simulink model "mldemo_suspn"  (Simulink 6.6)
settings: Solver=ode45  SolverMode=SingleTasking  StartTime=0.0  StopTime=10  MaxStep=0.01  RelTol=1e-3  AbsTol=1e-6
StopFcn:
  | pause(0.1)
  | mldemo_suspgraph
model workspace: external: M-Code (data not in the file)
values from neighbouring files (symbols this model uses):
  cf = cf0    (= 2200)    [configParams.m]    (also in myCostFcn.m = x(2); myCostFcnRR.m = x(2); mynonlcon.m = x(2); mynonlconRR.m = x(2))
  cr = cr0    (= 2000)    [configParams.m]    (also in myCostFcn.m = x(4); myCostFcnRR.m = x(4); mynonlcon.m = x(4); mynonlconRR.m = x(4))
  Iyy = Iyyempty    (= 2100)    [configParams.m]    (also in tweakmymass.m = Iyy1 - Mb*cm^2)
  kf = kf0    (= 19600)    [configParams.m]    (also in myCostFcn.m = x(1); myCostFcnRR.m = x(1); mynonlcon.m = x(1); mynonlconRR.m = x(1))
  kr = kr0    (= 14700)    [configParams.m]    (also in myCostFcn.m = x(3); myCostFcnRR.m = x(3); mynonlcon.m = x(3); mynonlconRR.m = x(3))
  Lf = Lf0    (= 0.9)    [configParams.m]    (also in tweakmymass.m = Lf0 - cm)
  Lr = Lr0    (= 1.2)    [configParams.m]    (also in tweakmymass.m = Lr0 + cm)
  Mb = Mempty    (= 1200)    [configParams.m]    (also in tweakmymass.m = Mempty + front + back + trunk)
  theta0 = 0    [configParams.m]
  thetadot0 = 0    [configParams.m]
  Z0 = -0.5*Mb*g/(kf+kr)    (= -0.171603498542)    [configParams.m]
  Zdot0 = 0    [configParams.m]
Description:
  | Automotive Suspension
  | 
  | This demo describes a simplified half-car model that includes an independent
  | front and rear vertical suspension. The model also includes body pitch and
  | bounce degrees of freedom. The demo provides a description of the model to
  | show how simulation can be used for investigating ride characteristics.
  | In conjunction with a powertrain simulation, the model could
  | investigate longitudinal shuffle resulting from changes in throttle setting.
settings Model: Creator=The MathWorks Inc.  LastModifiedBy=tschultz  ExtModeTrigMode=oneshot  ExtModeArmWhenConnect=off  ExtModeAutoUpdateStatusClock=off
settings DataIOCC: InitialState=x0  LimitDataPoints=off  SaveFormat=StructureWithTime  SaveOutput=off  StateSaveName=x  TimeSaveName=t  SignalLoggingName=sldemo_suspn_output
settings OptimizationCC: BooleanDataType=off  InlineInvariantSignals=on  BufferReusableBoundary=off
settings DebuggingCC: SignalResolutionControl=TryResolveAllWithWarning  SolverPrmCheckMsg=none  MultiTaskDSMMsg=warning  SigSpecEnsureSampleTimeMsg=none  IntegerOverflowMsg=none  BusObjectLabelMismatch=none  StrictBusMsg=ErrorLevel1
settings HardwareCC: TargetUnknown=on
settings RTWCC: IncludeERTFirstTime=on

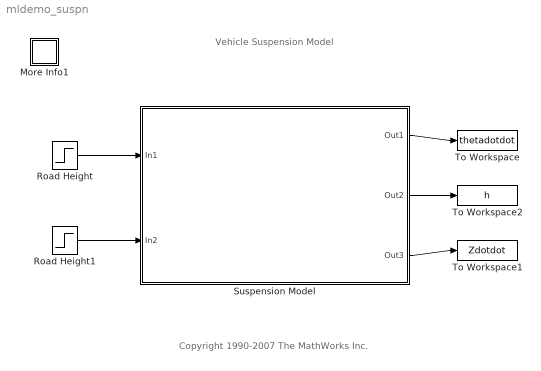
== system mldemo_suspn ==
  note: Vehicle Suspension Model
  note: Copyright 1990-2007 The MathWorks Inc.
  More Info1 : Subsystem
      settings: OpenFcn=showdemo(bdroot(gcb))
      mask Display: disp('?')
  Road Height : Step  After=0.01  SampleTime=0
  Road Height1 : Step  Time=2  After=-0.01  SampleTime=0
  Suspension Model : Subsystem
      mask Display: plot(-1, 0, 13, 12, [1 12], [11 11], [1 5], [2 2], [1 2], [4.5 5], [2 0], [5 6], [0 2], [6 7], [2 0], [7 8], [0 1], [8 8.5], [1 1], [8.5 11], [1 1], [2 4.5], [5 5], [2 5], [4 6], [5 5], [4 4], [5 8], [6 6], [5 8], [4 6], [6.5 6.5], [5 5], [6.5 11], [0 1], [1 2], [2 3], [1 2], [4 5], [1 2])
  To Workspace : ToWorkspace  VariableName=thetadotdot  SampleTime=-1  SaveFormat=Array
  To Workspace1 : ToWorkspace  VariableName=Zdotdot  SampleTime=-1  SaveFormat=Array
  To Workspace2 : ToWorkspace  VariableName=h  SampleTime=-1  SaveFormat=Array
  wires:
  Road Height/1 -> Suspension Model/1(In1)
  Road Height1/1 -> Suspension Model/2(In2)
  Suspension Model/1(Out1) -> To Workspace/1
  Suspension Model/2(Out2) -> To Workspace2/1
  Suspension Model/3(Out3) -> To Workspace1/1

== system mldemo_suspn/More Info1 ==

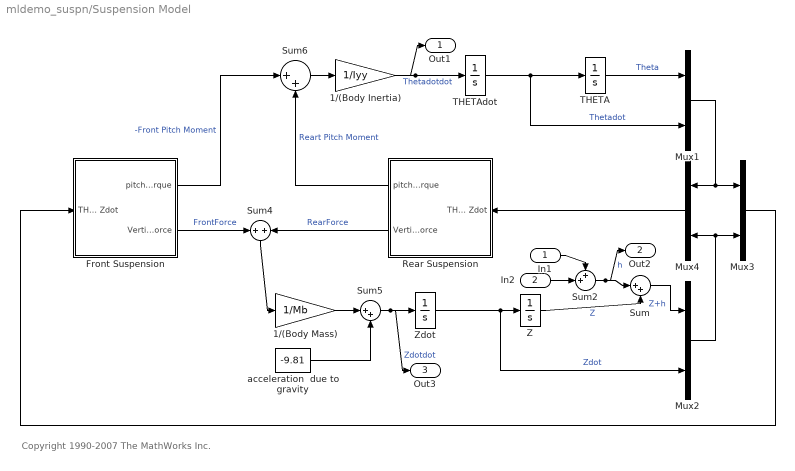
== system mldemo_suspn/Suspension Model ==
  note: Copyright 1990-2007 The MathWorks Inc.
  In1 : Inport
  In2 : Inport  Port=2
  1/(Body Inertia) : Gain  Gain=1/Iyy  SaturateOnIntegerOverflow=on
  1/(Body Mass) : Gain  Gain=1/Mb  SaturateOnIntegerOverflow=on
  Front Suspension : Subsystem  mask(half-car suspension){K=kf, C=cf, L=-Lf}
      mask prompts: K "Stiffness = spring rate:"; C "Damping rate:"; L "Moment arm:"
      mask help:
      | Half-Car Suspension
      | The spring and damping rates for an individual wheel are entered below.  Their combined effect as applied to two wheels at the specified distance from the center of mass is computed.  The distance should be specified as positive if the subsystem is oriented such that increasing z corresponds to increasing theta, negative otherwise.
      mask Help: See "Using Simulink and Stateflow in Automotive Applications" for a mathematical derivation of the subsystem operation.  Contact your MathWorks distributor to obtain a copy.
      mask Display: plot(-1, 0, 13, 12, [1 12], [11 11], [1 5], [2 2], [1 2], [4.5 5], [2 0], [5 6], [0 2], [6 7], [2 0], [7 8], [0 1], [8 8.5], [1 1], [8.5 11], [1 1], [2 4.5], [5 5], [2 5], [4 6], [5 5], [4 4], [5 8], [6 6], [5 8], [4 6], [6.5 6.5], [5 5], [6.5 11], [0 1], [1 2], [2 3], [1 2], [4 5], [1 2])
  Mux1 : Mux  Inputs=2
      settings: DisplayOption=signals
  Mux2 : Mux  Inputs=2
      settings: DisplayOption=signals
  Mux3 : Mux  Inputs=2
      settings: DisplayOption=signals
  Mux4 : Mux  Orientation=left  Inputs=2
      settings: DisplayOption=signals
  Rear Suspension : Subsystem  Orientation=left  mask(half-car suspension){K=kr, C=cr, L=Lr}
      mask prompts: K "Stiffness = spring rate:"; C "Damping rate:"; L "Moment arm:"
      mask help:
      | Half-Car Suspension
      | The spring and damping rates for an individual wheel are entered below.  Their combined effect as applied to two wheels at the specified distance from the center of mass is computed.  The distance should be specified as positive if the subsystem is oriented such that increasing z corresponds to increasing theta, negative otherwise.
      mask Help: See "Using Simulink and Stateflow in Automotive Applications" for a mathematical derivation of the subsystem operation.  Contact your MathWorks distributor to obtain a copy.
      mask Display: plot(-1, 0, 13, 12, [1 12], [11 11], [1 5], [2 2], [1 2], [4.5 5], [2 0], [5 6], [0 2], [6 7], [2 0], [7 8], [0 1], [8 8.5], [1 1], [8.5 11], [1 1], [2 4.5], [5 5], [2 5], [4 6], [5 5], [4 4], [5 8], [6 6], [5 8], [4 6], [6.5 6.5], [5 5], [6.5 11], [0 1], [1 2], [2 3], [1 2], [4 5], [1 2])
  Sum : Sum  Inputs=|++
  Sum2 : Sum  Inputs=++|
  Sum4 : Sum  Orientation=down  SaturateOnIntegerOverflow=on  InputSameDT=on
  Sum5 : Sum  Inputs=|++  SaturateOnIntegerOverflow=on  InputSameDT=on
  Sum6 : Sum  Inputs=|++  SaturateOnIntegerOverflow=on  InputSameDT=on
  THETA : Integrator  InitialCondition=theta0  ContinuousStateAttributes='theta'
  THETAdot : Integrator  InitialCondition=thetadot0  ContinuousStateAttributes='thetadot'
  Z : Integrator  InitialCondition=Z0  ContinuousStateAttributes='Z'
  Zdot : Integrator  InitialCondition=Zdot0  ContinuousStateAttributes='Zdot'
  acceleration  due to gravity : Constant  Value=-9.81
  Out1 : Outport
  Out2 : Outport  Port=2
  Out3 : Outport  Port=3
  wires:
  Front Suspension/2(Vertical Force) -> Sum4/1  "FrontForce"
  Rear Suspension/2(Vertical Force) -> Sum4/2  "RearForce"
  Sum4/1 -> 1/(Body Mass)/1
  Mux1/1 -> Mux3/1, Mux4/1
  Mux3/1 -> Front Suspension/1(THETA THETAdot Z Zdot)
  Mux4/1 -> Rear Suspension/1(THETA THETAdot Z Zdot)
  Sum5/1 -> Zdot/1, Out3/1  "Zdotdot"
  acceleration  due to gravity/1 -> Sum5/2
  1/(Body Mass)/1 -> Sum5/1
  Zdot/1 -> Z/1, Mux2/2  "Zdot"
  Sum6/1 -> 1/(Body Inertia)/1
  Rear Suspension/1(pitch Torque) -> Sum6/2  "Reart Pitch Moment"
  1/(Body Inertia)/1 -> Out1/1, THETAdot/1  "Thetadotdot"
  THETA/1 -> Mux1/1  "Theta"
  THETAdot/1 -> THETA/1, Mux1/2  "Thetadot"
  Mux2/1 -> Mux4/2, Mux3/2
  Sum2/1 -> Sum/1, Out2/1  "h"
  Z/1 -> Sum/2  "Z"
  Sum/1 -> Mux2/1  "Z+h"
  Front Suspension/1(pitch Torque) -> Sum6/1  "-Front Pitch Moment"
  In1/1 -> Sum2/1
  In2/1 -> Sum2/2

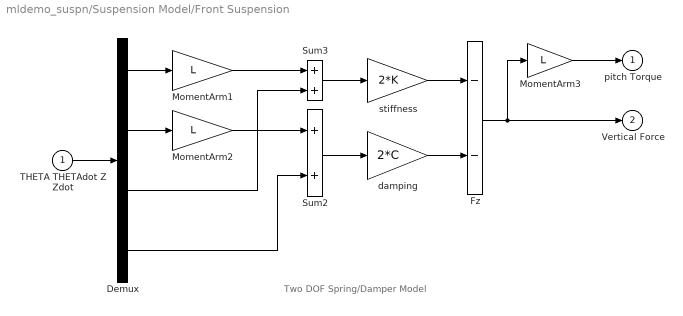
== system mldemo_suspn/Suspension Model/Front Suspension ==
  note: Two DOF Spring/Damper Model
  THETA THETAdot Z Zdot : Inport
  Demux : Demux
  Fz : Sum  Inputs=--  SaturateOnIntegerOverflow=on  InputSameDT=on
  MomentArm1 : Gain  Gain=L  SaturateOnIntegerOverflow=on
  MomentArm2 : Gain  Gain=L  SaturateOnIntegerOverflow=on
  MomentArm3 : Gain  Gain=L  SaturateOnIntegerOverflow=on
  Sum2 : Sum  SaturateOnIntegerOverflow=on  InputSameDT=on
  Sum3 : Sum  SaturateOnIntegerOverflow=on  InputSameDT=on
  damping : Gain  Gain=2*C  SaturateOnIntegerOverflow=on
  stiffness : Gain  Gain=2*K  SaturateOnIntegerOverflow=on
  pitch Torque : Outport
  Vertical Force : Outport  Port=2
  wires:
  Sum2/1 -> damping/1
  Sum3/1 -> stiffness/1
  THETA THETAdot Z Zdot/1 -> Demux/1
  damping/1 -> Fz/2
  stiffness/1 -> Fz/1
  Fz/1 -> Vertical Force/1, MomentArm3/1
  MomentArm3/1 -> pitch Torque/1
  Demux/1 -> MomentArm1/1
  Demux/2 -> MomentArm2/1
  Demux/3 -> Sum3/2
  MomentArm1/1 -> Sum3/1
  MomentArm2/1 -> Sum2/1
  Demux/4 -> Sum2/2

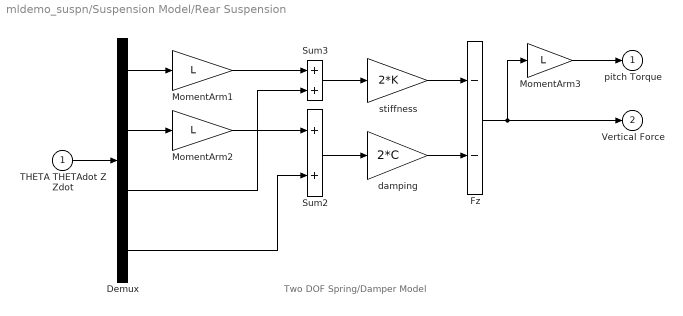
== system mldemo_suspn/Suspension Model/Rear Suspension ==
  note: Two DOF Spring/Damper Model
  THETA THETAdot Z Zdot : Inport
  Demux : Demux
  Fz : Sum  Inputs=--  SaturateOnIntegerOverflow=on  InputSameDT=on
  MomentArm1 : Gain  Gain=L  SaturateOnIntegerOverflow=on
  MomentArm2 : Gain  Gain=L  SaturateOnIntegerOverflow=on
  MomentArm3 : Gain  Gain=L  SaturateOnIntegerOverflow=on
  Sum2 : Sum  SaturateOnIntegerOverflow=on  InputSameDT=on
  Sum3 : Sum  SaturateOnIntegerOverflow=on  InputSameDT=on
  damping : Gain  Gain=2*C  SaturateOnIntegerOverflow=on
  stiffness : Gain  Gain=2*K  SaturateOnIntegerOverflow=on
  pitch Torque : Outport
  Vertical Force : Outport  Port=2
  wires:
  Demux/4 -> Sum2/2
  MomentArm2/1 -> Sum2/1
  MomentArm1/1 -> Sum3/1
  Demux/3 -> Sum3/2
  Demux/2 -> MomentArm2/1
  Demux/1 -> MomentArm1/1
  MomentArm3/1 -> pitch Torque/1
  Fz/1 -> MomentArm3/1, Vertical Force/1
  stiffness/1 -> Fz/1
  damping/1 -> Fz/2
  THETA THETAdot Z Zdot/1 -> Demux/1
  Sum3/1 -> stiffness/1
  Sum2/1 -> damping/1
